simulink model "T3_Linarized_VS_NonLin_2_dof_Helicopter"  (R2023a)
settings: Solver=ode4  StartTime=0.0  StopTime=inf  FixedStep=0.1  RelTol=1e-3
values from neighbouring files (symbols this model uses):
  Ac = [0,0,1,0 ... (first row only)    [Linerized_Parameters.m]
  B_p = 0.01    [Heli_Parameters.m]
  B_y = 0.08    [Heli_Parameters.m]
  Bc = [0,0 ... (first row only)    [Linerized_Parameters.m]
  g = 9.81    [Heli_Parameters.m]
  J_eqp = 0.0172    [Heli_Parameters.m]
  J_eqy = 0.0210    (= 0.021)    [Heli_Parameters.m]
  K_pp = 0.0556    [Heli_Parameters.m]
  K_py = 0.005    [Heli_Parameters.m]
  K_yp = 0.15    [Heli_Parameters.m]
  K_yy = 0.21084    [Heli_Parameters.m]
  l_cm = 0.015    [Heli_Parameters.m]
  m_heli = 0.479    [Heli_Parameters.m]
  p_op = pi/2    (= 1.57079632679)    [Linerized_Parameters.m]
  t_op = (-10*pi)/180    (= -0.174532925199)    [Linerized_Parameters.m]
  V_mp_op = (K_yy* m_heli*g*cos(t_op)*l_cm  )/((K_yy*K_pp-K_yp*K_py))    [Linerized_Parameters.m]
  V_my_op = (K_yp* V_mp_op)/K_yy    [Linerized_Parameters.m]
  wp_op = 0    [Linerized_Parameters.m]
  wt_op = 0    [Linerized_Parameters.m]
libraries: realtime_pacer_lib x1
settings Model: Creator=aleho  LastModifiedBy=aleho

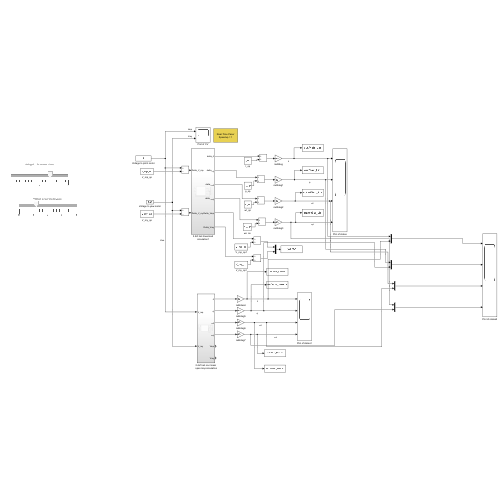
[thumbnail: Simulink's stored preview of the top-level diagram]
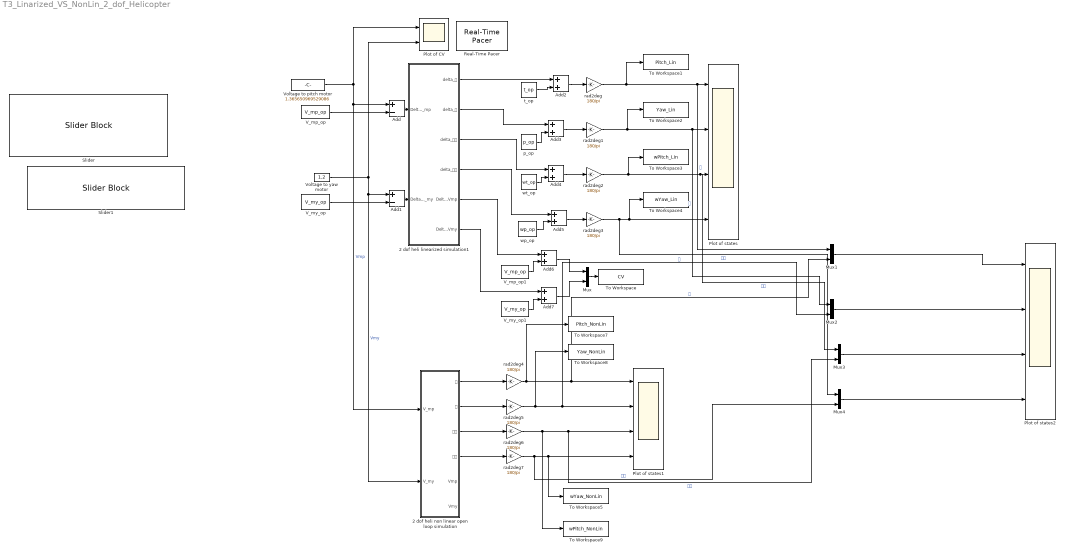
== system T3_Linarized_VS_NonLin_2_dof_Helicopter ==
  2 dof heli linearized simulation1 : Subsystem
  2 dof heli non linear open loop simulation : Subsystem
  Add : Sum  Inputs=+-
  Add1 : Sum  Inputs=+-
  Add{2..7} (6 alike) : Sum
  Mux{,1..4} (5 alike) : Mux  Inputs=2
  Plot of CV : Scope  NumInputPorts=2
  Plot of states : Scope  NumInputPorts=4
  Plot of states1 : Scope  NumInputPorts=4
  Plot of states2 : Scope  NumInputPorts=4
  Real-Time Pacer : realtime_pacer_lib/Real-Time Pacer  simTimePerRealTime=1
  Slider : SliderBlock  ScaleMax=2  TickInterval=1
  Slider1 : SliderBlock  ScaleMax=4  TickInterval=1
  To Workspace : ToWorkspace  VariableName=CV  SaveFormat=Timeseries  SampleTime=-1
  To Workspace1 : ToWorkspace  VariableName=Pitch_Lin  SaveFormat=Timeseries  SampleTime=-1
  To Workspace2 : ToWorkspace  VariableName=Yaw_Lin  SaveFormat=Timeseries  SampleTime=-1
  To Workspace3 : ToWorkspace  VariableName=wPitch_Lin  SaveFormat=Timeseries  SampleTime=-1
  To Workspace4 : ToWorkspace  VariableName=wYaw_Lin  SaveFormat=Timeseries  SampleTime=-1
  To Workspace5 : ToWorkspace  VariableName=wYaw_NonLin  SaveFormat=Timeseries  SampleTime=-1
  To Workspace7 : ToWorkspace  VariableName=Pitch_NonLin  SaveFormat=Timeseries  SampleTime=-1
  To Workspace8 : ToWorkspace  VariableName=Yaw_NonLin  SaveFormat=Timeseries  SampleTime=-1
  To Workspace9 : ToWorkspace  VariableName=wPitch_NonLin  SaveFormat=Timeseries  SampleTime=-1
  V_mp_op : Constant  Value=V_mp_op
  V_mp_op1 : Constant  Value=V_mp_op
  V_my_op : Constant  Value=V_my_op
  V_my_op1 : Constant  Value=V_my_op
  Voltage to pitch motor : Constant  Value=1.365650969529086
  Voltage to yaw motor : Constant  Value=1.2
  p_op : Constant  Value=p_op
  rad2deg{,1..7} (8 alike) : Gain  Gain=180/pi
  t_op : Constant  Value=t_op
  wp_op : Constant  Value=wp_op
  wt_op : Constant  Value=wt_op
  wires:
  Voltage to pitch motor/1 -> 2 dof heli non linear open loop simulation/1(V_mp), Add/1, Plot of CV/1  "Vmp"
  Voltage to yaw motor/1 -> Plot of CV/2, Add1/1, 2 dof heli non linear open loop simulation/2(V_my)  "Vmy"
  Add/1 -> 2 dof heli linearized simulation1/1(Delta_V_mp)
  V_mp_op/1 -> Add/2
  Add1/1 -> 2 dof heli linearized simulation1/2(Delta_V_my)
  V_my_op/1 -> Add1/2
  t_op/1 -> Add2/2
  p_op/1 -> Add3/2
  wp_op/1 -> Add5/2
  wt_op/1 -> Add4/2
  2 dof heli linearized simulation1/1(delta_𝜃) -> Add2/1
  2 dof heli linearized simulation1/2(delta_𝜓) -> Add3/1
  2 dof heli linearized simulation1/3(delta_𝜔𝜃) -> Add4/1
  2 dof heli linearized simulation1/4(delta_𝜔𝜓) -> Add5/1
  rad2deg/1 -> To Workspace1/1, Mux1/1, Plot of states/1  "𝜃"
  Add2/1 -> rad2deg/1
  rad2deg1/1 -> To Workspace2/1, Mux2/1, Plot of states/2  "𝜓"
  Add3/1 -> rad2deg1/1
  rad2deg2/1 -> To Workspace3/1, Mux3/1, Plot of states/3  "𝜔𝜃"
  Add4/1 -> rad2deg2/1
  rad2deg3/1 -> Mux4/1, To Workspace4/1, Plot of states/4  "𝜔𝜓"
  Add5/1 -> rad2deg3/1
  2 dof heli linearized simulation1/5(Delta_Vmp) -> Add6/1
  Add6/1 -> Mux/1
  2 dof heli linearized simulation1/6(Delta_Vmy) -> Add7/1
  Add7/1 -> Mux/2
  V_mp_op1/1 -> Add6/2
  V_my_op1/1 -> Add7/2
  Mux/1 -> To Workspace/1
  2 dof heli non linear open loop simulation/2(𝜓) -> rad2deg5/1
  2 dof heli non linear open loop simulation/3(𝜔𝜃) -> rad2deg6/1
  2 dof heli non linear open loop simulation/4(𝜔𝜓) -> rad2deg7/1
  2 dof heli non linear open loop simulation/1(𝜃) -> rad2deg4/1
  rad2deg7/1 -> Mux4/2, To Workspace5/1, Plot of states1/4  "𝜔𝜓"
  rad2deg4/1 -> To Workspace7/1, Mux1/2, Plot of states1/1  "𝜃"
  rad2deg6/1 -> To Workspace9/1, Mux3/2, Plot of states1/3  "𝜔𝜃"
  rad2deg5/1 -> To Workspace8/1, Mux2/2, Plot of states1/2  "𝜓"
  Mux1/1 -> Plot of states2/1
  Mux2/1 -> Plot of states2/2
  Mux3/1 -> Plot of states2/3
  Mux4/1 -> Plot of states2/4

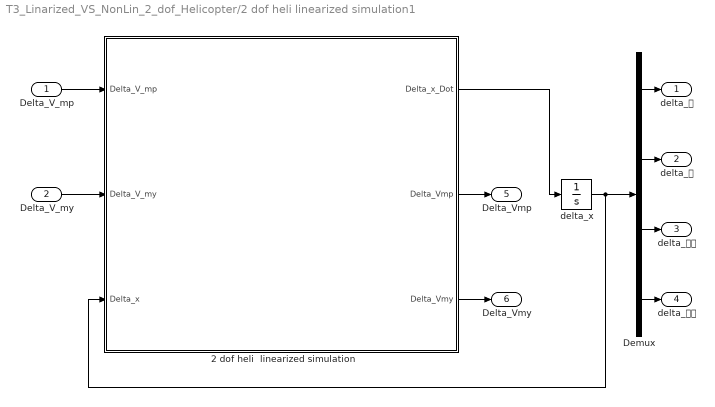
== system T3_Linarized_VS_NonLin_2_dof_Helicopter/2 dof heli linearized simulation1 ==
  Delta_V_mp : Inport
  Delta_V_my : Inport  Port=2
  2 dof heli  linearized simulation : MATLAB Function  TreatAsAtomicUnit=on
  Demux : Demux
  delta_x : Integrator  InitialCondition=[-45*pi/180,pi/2,0,0]  LimitOutput=on  UpperSaturationLimit=[45*pi/180-t_op,pi+p_op,2,2]  LowerSaturationLimit=[-45*pi/180+t_op,0-p_op,-2,-2]
  delta_𝜃 : Outport
  delta_𝜓 : Outport  Port=2
  delta_𝜔𝜃 : Outport  Port=3
  delta_𝜔𝜓 : Outport  Port=4
  Delta_Vmp : Outport  Port=5
  Delta_Vmy : Outport  Port=6
  wires:
  Delta_V_mp/1 -> 2 dof heli  linearized simulation/1(Delta_V_mp)
  delta_x/1 -> 2 dof heli  linearized simulation/3(Delta_x), Demux/1
  Demux/1 -> delta_𝜃/1
  Demux/4 -> delta_𝜔𝜓/1
  Demux/3 -> delta_𝜔𝜃/1
  Demux/2 -> delta_𝜓/1
  2 dof heli  linearized simulation/1(Delta_x_Dot) -> delta_x/1
  Delta_V_my/1 -> 2 dof heli  linearized simulation/2(Delta_V_my)
  2 dof heli  linearized simulation/2(Delta_Vmp) -> Delta_Vmp/1
  2 dof heli  linearized simulation/3(Delta_Vmy) -> Delta_Vmy/1

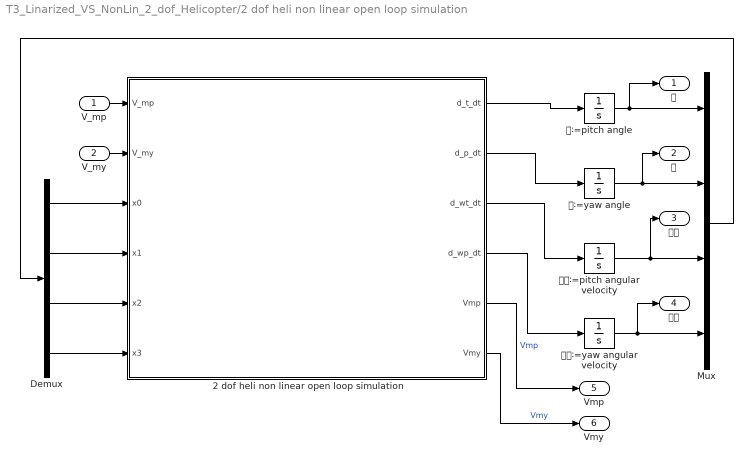
== system T3_Linarized_VS_NonLin_2_dof_Helicopter/2 dof heli non linear open loop simulation ==
  V_mp : Inport
  V_my : Inport  Port=2
  2 dof heli non linear open loop simulation : MATLAB Function  TreatAsAtomicUnit=on
  Demux : Demux
  Mux : Mux
  𝜃∶=pitch angle : Integrator  InitialCondition=-10*pi/180  LimitOutput=on  UpperSaturationLimit=45*pi/180  LowerSaturationLimit=-45*pi/180
  𝜓∶=yaw angle : Integrator  InitialCondition=pi/2  LimitOutput=on  UpperSaturationLimit=pi  LowerSaturationLimit=0
  𝜔𝜃∶=pitch angular velocity : Integrator  LimitOutput=on  UpperSaturationLimit=2*pi  LowerSaturationLimit=-2*pi
  𝜔𝜓∶=yaw angular velocity : Integrator  LimitOutput=on  UpperSaturationLimit=2*pi  LowerSaturationLimit=-2*pi
  𝜃 : Outport
  𝜓 : Outport  Port=2
  𝜔𝜃 : Outport  Port=3
  𝜔𝜓 : Outport  Port=4
  Vmp : Outport  Port=5
  Vmy : Outport  Port=6
  wires:
  V_mp/1 -> 2 dof heli non linear open loop simulation/1(V_mp)
  𝜔𝜃∶=pitch angular velocity/1 -> 𝜔𝜃/1, Mux/3
  Demux/4 -> 2 dof heli non linear open loop simulation/6(x3)
  𝜔𝜓∶=yaw angular velocity/1 -> 𝜔𝜓/1, Mux/4
  Mux/1 -> Demux/1
  𝜃∶=pitch angle/1 -> 𝜃/1, Mux/1
  𝜓∶=yaw angle/1 -> 𝜓/1, Mux/2
  2 dof heli non linear open loop simulation/1(d_t_dt) -> 𝜃∶=pitch angle/1
  V_my/1 -> 2 dof heli non linear open loop simulation/2(V_my)
  Demux/1 -> 2 dof heli non linear open loop simulation/3(x0)
  Demux/3 -> 2 dof heli non linear open loop simulation/5(x2)
  Demux/2 -> 2 dof heli non linear open loop simulation/4(x1)
  2 dof heli non linear open loop simulation/2(d_p_dt) -> 𝜓∶=yaw angle/1
  2 dof heli non linear open loop simulation/4(d_wp_dt) -> 𝜔𝜓∶=yaw angular velocity/1
  2 dof heli non linear open loop simulation/3(d_wt_dt) -> 𝜔𝜃∶=pitch angular velocity/1
  2 dof heli non linear open loop simulation/5(Vmp) -> Vmp/1  "Vmp"
  2 dof heli non linear open loop simulation/6(Vmy) -> Vmy/1  "Vmy"

== matlab function T3_Linarized_VS_NonLin_2_dof_Helicopter/2 dof heli linearized simulation1/2 dof heli  linearized simulation ==
  data: Delta_V_mp input; Delta_V_my input; Delta_x input; Bc parameter; Ac parameter; Delta_x_Dot output; Delta_Vmp output; Delta_Vmy output
function [Delta_x_Dot, Delta_Vmp,Delta_Vmy] = linear_model(Delta_V_mp,Delta_V_my,Delta_x, Bc, Ac)

Delta_Vmp = Delta_V_mp;
Delta_Vmy = Delta_V_my;

% Linear state space model equation
Delta_u = [Delta_V_mp ;Delta_V_my];
Delta_x_Dot = Ac*Delta_x + Bc*Delta_u;

== matlab function T3_Linarized_VS_NonLin_2_dof_Helicopter/2 dof heli non linear open loop simulation/2 dof heli non linear open loop simulation ==
  data: V_mp input; V_my input; d_t_dt output; d_p_dt output; d_wt_dt output; d_wp_dt output; x0 input; x1 input; x2 input; x3 input; l_cm parameter; m_heli parameter; J_eqp parameter; J_eqy parameter; g parameter; K_pp parameter; K_yy parameter; K_py parameter; K_yp parameter; B_p parameter; B_y parameter; Vmp output; Vmy output
function [d_t_dt,d_p_dt,d_wt_dt,d_wp_dt, Vmp,Vmy] =  heli_2_dof_ODE_eqs(V_mp,V_my,x0,x1,x2,x3,l_cm, m_heli, J_eqp, J_eqy, g, K_pp, K_yy, K_py, K_yp, B_p, B_y)
% States
t = x0;    % pitch angle ( theta )
p = x1;    % yaw angle ( psi )
wt = x2;   % pitch angular velocity ( Omega theta )
wp = x3;   % yaw angular velocity ( Omega psi )

% Control voltages
Vmp = V_mp;
Vmy = V_my;

% ODEs
% pitch angle
d_t_dt = wt;

% yaw angle
d_p_dt = wp;

% pitch angular velocity
d_wt_dt = ((K_pp*V_mp)/(J_eqp+m_heli*l_cm^2)) - ((K_py*V_my)/(J_eqp+m_heli*l_cm^2))...
    - ((B_p*wt+m_heli*wp^2*sin(t)*l_cm^2*cos(t)+m_heli*g*cos(t)*l_cm) / (J_eqp+m_heli*l_cm^2));

% yaw angular velocity
d_wp_dt = ((K_yp*V_mp)/(J_eqy+m_heli*cos(t)^2*l_cm^2)) -...
    ((K_yy*V_my)/(J_eqy+m_heli*cos(t)^2*l_cm^2)) +...
    ((2*m_heli*wp*sin(t)*l_cm^2*cos(t)*wt)/(J_eqy+m_heli*cos(t)^2*l_cm^2))...
    - ((B_y*wp)/(J_eqy+m_heli*cos(t)^2*l_cm^2));
